simulink model "preg2"  (R2021a)
settings: Solver=VariableStepAuto  StartTime=0.0  StopTime=10.0  RelTol=1e-3
settings Model: Creator=Felipe  LastModifiedBy=Felipe

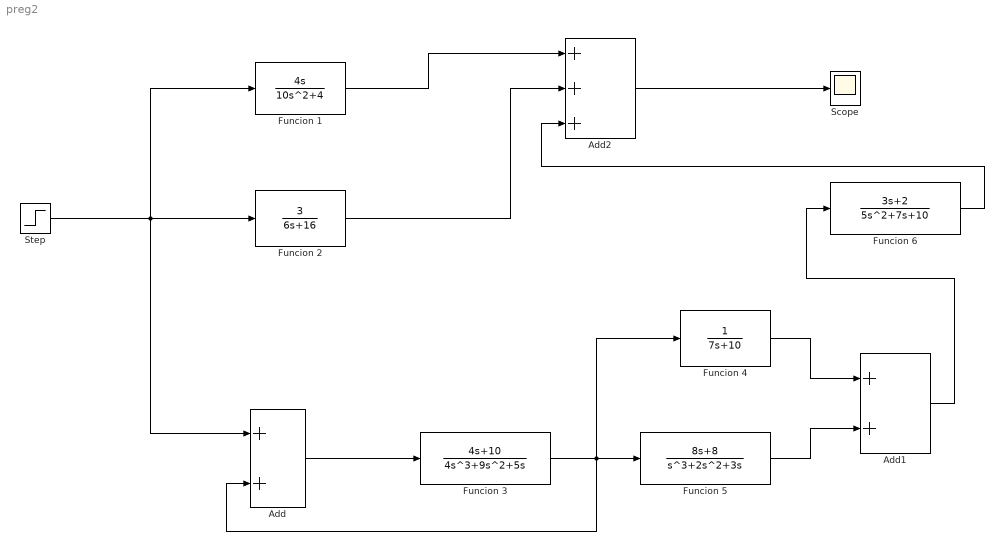
== system preg2 ==
  Add : Sum
  Add1 : Sum
  Add2 : Sum  Inputs=+++
  Funcion 1 : TransferFcn  Numerator=[4 0]  Denominator=[10 0 4]
  Funcion 2 : TransferFcn  Numerator=[3]  Denominator=[6 16]
  Funcion 3 : TransferFcn  Numerator=[4 10]  Denominator=[4 9 5 0]
  Funcion 4 : TransferFcn  Denominator=[7 10]
  Funcion 5 : TransferFcn  Numerator=[8 8]  Denominator=[1 2 3 0]
  Funcion 6 : TransferFcn  Numerator=[3 2]  Denominator=[5 7 10]
  Scope : Scope
  Step : Step  Time=0  SampleTime=0
  wires:
  Add/1 -> Funcion 3/1
  Funcion 4/1 -> Add1/1
  Funcion 5/1 -> Add1/2
  Add1/1 -> Funcion 6/1
  Funcion 1/1 -> Add2/1
  Funcion 2/1 -> Add2/2
  Funcion 6/1 -> Add2/3
  Add2/1 -> Scope/1
  Funcion 3/1 -> Add/2, Funcion 5/1, Funcion 4/1
  Step/1 -> Funcion 1/1, Funcion 2/1, Add/1
